simulink model "Linear_PID_TDSO_MODEL"  (Simulink 7.6)
settings: Solver=ode45  StartTime=0.0  StopTime=20  RelTol=1e-3
libraries: ADRC x1
settings Model: Creator=Administrator  LastModifiedBy=Administrator
settings DebuggingCC: SolverPrmCheckMsg=none

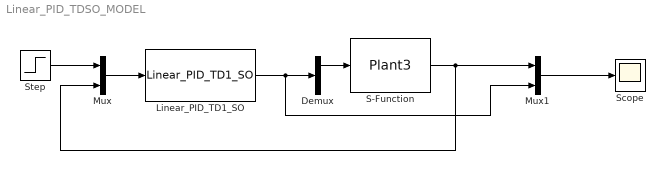
== system Linear_PID_TDSO_MODEL ==
  Demux : Demux  Outputs=2
  Linear_PID_TD1_SO : ADRC/LinearPID/Linear_PID_TD1_SO  r0=1  h=0.004  B=[100,300]  Bet=[30,50,20]  D=0.02
  Mux : Mux  Inputs=2
  Mux1 : Mux  Inputs=2
  S-Function : S-Function  FunctionName=Plant3  EnableBusSupport=off
  Scope : Scope
      settings: YMax=2
  Step : Step  Time=0  After=1.5  SampleTime=0
  wires:
  Step/1 -> Mux/1
  Mux/1 -> Linear_PID_TD1_SO/1
  Mux1/1 -> Scope/1
  Linear_PID_TD1_SO/1 -> Demux/1, Mux1/2
  Demux/1 -> S-Function/1
  S-Function/1 -> Mux1/1, Mux/2
